simulink library "libopencn"  (R2019b)
settings: Solver=VariableStepAuto  StartTime=0.0  StopTime=10.0  RelTol=1e-3
settings Model: Creator=peter  LastModifiedBy=peter
settings RTWCC: RTWUseSimCustomCode=on  TargetLang=C++
settings GRTTargetCC: TargetLangStandard=C++03 (ISO)  MultiInstanceERTCode=on  CodeInterfacePackaging=C++ class

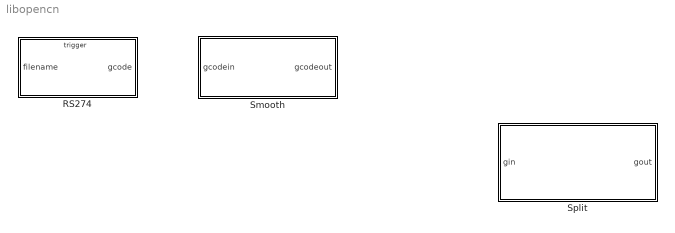
== system libopencn ==
  "RS274 " : Stateflow chart  BlockKeywords=__PRM__SERIALIZED__DATA__:Stateflow Chart,Stateflow Diagram  TreatAsAtomicUnit=on
  Smooth : Stateflow chart  BlockKeywords=__PRM__SERIALIZED__DATA__:Stateflow Chart,Stateflow Diagram  TreatAsAtomicUnit=on
  Split : Stateflow chart  BlockKeywords=__PRM__SERIALIZED__DATA__:Stateflow Chart,Stateflow Diagram  TreatAsAtomicUnit=on

== stateflow chart libopencn/RS274  ==
  settings: executeAtInitialization=1
  state Start
  state Load
    [status, curv] = ReadGCode(ReadGCodeCmd.Load, char(filename));
    curv = ConstrLineStruct([1,2,3]', [4,5,6]', 0.7, ZSpdMode.NN);
    curv.Type = CurveType.None;
  state End
    entry:
    curv.Type = CurveType.None;
    gcode.data = curv;
    send(gcode);
  state Read
    [status, curv] = ReadGCode(ReadGCodeCmd.Read, '');
    if curv.Type ~= CurveType.None
    gcode.data = curv;
    send(gcode);
    end
  (default) -> Start
  Start -> Load
  Load -> End [order 2] : [status == 0]
  Load -> Read [order 1] : [status == 1]
  Read -> End : [status == 0]
  data: gcode output Bus: CurvStruct; status local int32 size=1 =int32(0); curv local Bus: CurvStruct size=1; filename input =""
  events: read input FUNCTION_CALL_EVENT

== stateflow chart libopencn/Split ==
  state Start
  state Stop
    entry:
    curv_structs = SplitCurvStruct(gin.data, 2.0);
    for k = 1:length(curv_structs)
    gout.data = curv_structs(k);
    send(gout);
    end
  state End
  (default) -> Start
  Start -> Stop [order 1] : gin[gin.data.Type ~= 0]
  Start -> End [order 2] : gin
  Stop -> Stop [order 1] : gin[gin.data.Type ~= 0]
  Stop -> End [order 2] : gin
  data: gin input Bus: CurvStruct; gout output Bus: CurvStruct; k local; curv_structs local Bus: CurvStruct

== stateflow chart libopencn/Smooth ==
  state Start
  state FirstReceive
    entry:
    C2 = gcodein.data
  state Receive
    entry:
    gcode = gcodein.data;
    [C1, CT, C2] = CalcTransition(C2, gcode, 0.2);
    gcodeout.data = C1;
    send(gcodeout);
    gcodeout.data = CT;
    send(gcodeout);
  state End
  state SendLast
    entry:
    gcodeout.data = C2;
    send(gcodeout);
  (default) -> Start
  Start -> FirstReceive : gcodein
  FirstReceive -> SendLast [order 2] : gcodein
  FirstReceive -> Receive [order 1] : gcodein[gcodein.data.Type ~= 0]
  Receive -> Receive [order 1] : gcodein[gcodein.data.Type ~= 0]
  SendLast -> End
  Receive -> SendLast [order 2] : gcodein
  data: gcodein input Bus: CurvStruct size=1; gcodeout output Bus: CurvStruct; C1 local Bus: CurvStruct; C2 local Bus: CurvStruct; CT local Bus: CurvStruct; gcode local Bus: CurvStruct
